simulink model "sistema_mecanico_lagrange"  (R2018a)
settings: Solver=VariableStepAuto  StartTime=0.0  StopTime=2  RelTol=1e-3
settings Model: Creator=carma  LastModifiedBy=carma

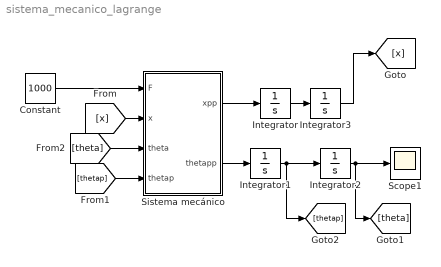
== system sistema_mecanico_lagrange ==
  Constant : Constant  Value=1000
  Integrator{,1..3} (4 alike) : Integrator
  Scope1 : Scope
  Sistema mecánico : MATLAB Function  TreatAsAtomicUnit=on
  wires:
  Constant/1 -> Sistema mecánico/1(F)
  Sistema mecánico/1(xpp) -> Integrator/1
  Sistema mecánico/2(thetapp) -> Integrator1/1
  Integrator1/1 -> [thetap], Integrator2/1
  Integrator/1 -> Integrator3/1
  Integrator3/1 -> [x]
  [x] -> Sistema mecánico/2(x)
  Integrator2/1 -> [theta], Scope1/1
  [thetap] -> Sistema mecánico/4(thetap)
  [theta] -> Sistema mecánico/3(theta)

== matlab function sistema_mecanico_lagrange/Sistema mecánico ==
  data: F input; xpp output; x input; theta input; thetap input; thetapp output
function [xpp,thetapp] = fcn(F,x,theta, thetap)

%Parametros oscilaciones
r=0.01;
M=10;
k1=15;
k2=25;
k=10;
J=0.1;
b=2;



%ecuaciones dinámicas
xpp=(-k1*x-k2*(x-r*theta))/M;
thetapp=(F*r-k*theta-k2*r*(r*theta-x)-b*thetap)/J;
